simulink model "RefModel_SensorFault"  (R2020a)
settings: Solver=ode1  StartTime=0.0  StopTime=10.0  FixedStep=Ts_SensorFault.Ts_base  RelTol=1e-3
settings Model: Creator=sl  LastModifiedBy=Administrator
settings OptimizationCC: DefaultParameterBehavior=Inlined  EnhancedBackFolding=on  PassReuseOutputArgsAs=Individual arguments  ZeroExternalMemoryAtStartup=off  ZeroInternalMemoryAtStartup=off  OptimizeBlockOrder=speed  DifferentSizesBufferReuse=on  OptimizationCustomize=off  EfficientTunableParamExpr=on
settings DebuggingCC: InheritedTsInSrcMsg=none  ParameterPrecisionLossMsg=none  ParameterTunabilityLossMsg=error  UnconnectedInputMsg=none  UnconnectedOutputMsg=none  UnconnectedLineMsg=none
settings HardwareCC: ProdBitPerPointer=32  ProdBitPerSizeT=32  ProdBitPerPtrDiffT=32  ProdLargestAtomicInteger=Long  ProdLargestAtomicFloat=Double  ProdWordSize=32  ProdHWDeviceType=ARM Compatible->ARM Cortex
settings ModelReferenceCC: ModelReferenceNumInstancesAllowed=Single
settings SFSimCC: MATLABDynamicMemAlloc=off
settings RTWCC: SystemTargetFile=ert.tlc  TemplateMakefile=ert_default_tmf  GenerateReport=on  IncludeHyperlinkInReport=on  LaunchReport=on  GenerateTraceInfo=on  GenerateTraceReport=on  GenerateTraceReportSl=on  GenerateTraceReportSf=on  GenerateTraceReportEml=on
settings CodeAppCC: ForceParamTrailComments=on  IgnoreCustomStorageClasses=off  MaxIdLength=48  OperatorAnnotations=on  SimulinkDataObjDesc=on  SFDataObjDesc=on  InsertBlockDesc=on
settings ERTTargetCC: TargetLangStandard=C99 (ISO)  GenerateSampleERTMain=on  LogVarNameModifier=none  SupportVariableSizeSignals=on  InlinedParameterPlacement=NonHierarchical  ERTCustomFileTemplate=example_file_process.tlc

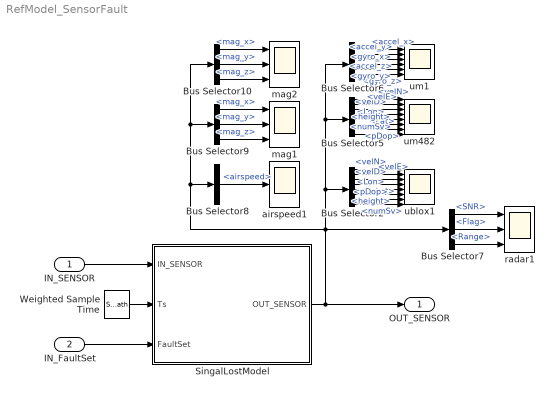
== system RefModel_SensorFault ==
  IN_SENSOR : Inport  OutDataTypeStr=Bus: BUS_SENSOR  BusOutputAsStruct=on
  IN_FaultSet : Inport  Port=2  OutDataTypeStr=Bus: BUS_SENSORFAULT_IN  BusOutputAsStruct=on
  Bus Selector10 : BusSelector  OutputSignals=mag2.mag_x,mag2.mag_y,mag2.mag_z
  Bus Selector2 : BusSelector  OutputSignals=ublox1.velN,ublox1.velE,ublox1.velD,ublox1.Lat,ublox1.Lon,ublox1.height,ublox1.pDop,ublox1.numSv
  Bus Selector5 : BusSelector  OutputSignals=um482.velN,um482.velE,um482.velD,um482.Lat,um482.Lon,um482.height,um482.pDop,um482.numSv
  Bus Selector6 : BusSelector  OutputSignals=IMU1.accel_x,IMU1.accel_y,IMU1.accel_z,IMU1.gyro_x,IMU1.gyro_y,IMU1.gyro_z
  Bus Selector7 : BusSelector  OutputSignals=radar1.SNR,radar1.Flag,radar1.Range
  Bus Selector8 : BusSelector  OutputSignals=airspeed1.airspeed
  Bus Selector9 : BusSelector  OutputSignals=mag1.mag_x,mag1.mag_y,mag1.mag_z
  SingalLostModel : Stateflow chart  TreatAsAtomicUnit=on
  Weighted Sample Time : SampleTimeMath  TsampMathOp=Ts Only
  airspeed1 : Scope
  mag1 : Scope  NumInputPorts=3
  mag2 : Scope  NumInputPorts=3
  radar1 : Scope  NumInputPorts=3
  ublox1 : Scope  NumInputPorts=8
  um1 : Scope  NumInputPorts=6
  um482 : Scope  NumInputPorts=8
  OUT_SENSOR : Outport  OutDataTypeStr=Bus: BUS_SENSOR  BusOutputAsStruct=on
  wires:
  Weighted Sample Time/1 -> SingalLostModel/2(Ts)
  IN_FaultSet/1 -> SingalLostModel/3(FaultSet)
  IN_SENSOR/1 -> SingalLostModel/1(IN_SENSOR)
  Bus Selector9/3 -> mag1/3  "<mag_z>"
  Bus Selector6/6 -> um1/6  "<gyro_z>"
  Bus Selector5/5 -> um482/5  "<Lon>"
  SingalLostModel/1(OUT_SENSOR) -> OUT_SENSOR/1, Bus Selector6/1, Bus Selector5/1, Bus Selector2/1, Bus Selector7/1, Bus Selector10/1, Bus Selector9/1, Bus Selector8/1
  Bus Selector6/4 -> um1/4  "<gyro_x>"
  Bus Selector6/2 -> um1/2  "<accel_y>"
  Bus Selector6/5 -> um1/5  "<gyro_y>"
  Bus Selector7/2 -> radar1/2  "<Flag>"
  Bus Selector5/3 -> um482/3  "<velD>"
  Bus Selector5/1 -> um482/1  "<velN>"
  Bus Selector5/4 -> um482/4  "<Lat>"
  Bus Selector5/8 -> um482/8  "<numSv>"
  Bus Selector7/3 -> radar1/3  "<Range>"
  Bus Selector5/7 -> um482/7  "<pDop>"
  Bus Selector2/1 -> ublox1/1  "<velN>"
  Bus Selector2/3 -> ublox1/3  "<velD>"
  Bus Selector2/4 -> ublox1/4  "<Lat>"
  Bus Selector6/1 -> um1/1  "<accel_x>"
  Bus Selector2/5 -> ublox1/5  "<Lon>"
  Bus Selector5/6 -> um482/6  "<height>"
  Bus Selector2/6 -> ublox1/6  "<height>"
  Bus Selector5/2 -> um482/2  "<velE>"
  Bus Selector2/8 -> ublox1/8  "<numSv>"
  Bus Selector2/2 -> ublox1/2  "<velE>"
  Bus Selector8/1 -> airspeed1/1  "<airspeed>"
  Bus Selector10/1 -> mag2/1  "<mag_x>"
  Bus Selector9/2 -> mag1/2  "<mag_y>"
  Bus Selector10/2 -> mag2/2  "<mag_y>"
  Bus Selector7/1 -> radar1/1  "<SNR>"
  Bus Selector6/3 -> um1/3  "<accel_z>"
  Bus Selector9/1 -> mag1/1  "<mag_x>"
  Bus Selector2/7 -> ublox1/7  "<pDop>"
  Bus Selector10/3 -> mag2/3  "<mag_z>"

== stateflow chart RefModel_SensorFault/SingalLostModel ==
  settings: executeAtInitialization=1
  state Others [parallel]
    settings: executionOrder=1
    state Normal
      du:
      OUT_SENSOR.time = IN_SENSOR.time;
    (default) -> Others.Normal
  state mag1 [parallel]
    en,du:
    sensorLocal = FaultSet.mag1;
    sensorDataLocal = IN_SENSOR.mag1;
    settings: executionOrder=9
    state Normal
      en:
      du:
      OUT_SENSOR.mag1 = sensorDataLocal;
    state Abnormal
      state SignalStuck
        % 信号保持最后有效值
        en:
        du:
      state SignalZero
        % 信号置零
        en,du:
        OUT_SENSOR.mag1 = setZero_mag(sensorDataLocal);
      state SignalDegrade
        % 信号精度降低
        en,du:
        OUT_SENSOR.mag1 = setDegrade_mag(sensorDataLocal);
      state SignalJump
        % 信号跳变
        en:
        tempJumpVal = 0.2*rand(1,3);
        on every((25+15*rand(1))/Ts,tick):
        tempJumpVal = 0.2*rand(1,3);
        du:
        OUT_SENSOR.mag1 = setJump_mag(sensorDataLocal,tempJumpVal);
      (default) -> mag1.Abnormal.SignalStuck
      (junction 486) -> mag1.Abnormal.SignalStuck : [whereToGo(sensorLocal) == ENUM_Fault.SingalStuck]
      (junction 488) -> (junction 486) [order 2]
      mag1.Abnormal.SignalStuck -> (junction 487) : [whereToGo(sensorLocal) ~= ENUM_Fault.SingalStuck]
      (junction 487) -> (junction 489)
      (junction 488) -> mag1.Abnormal.SignalZero [order 1] : [whereToGo(sensorLocal) == ENUM_Fault.SignalZero]
      (junction 490) -> (junction 488) [order 2]
      mag1.Abnormal.SignalZero -> (junction 489) : [whereToGo(sensorLocal) ~= ENUM_Fault.SignalZero]
      (junction 489) -> (junction 491)
      (junction 490) -> mag1.Abnormal.SignalDegrade [order 1] : [whereToGo(sensorLocal) == ENUM_Fault.SignalDegrade]
      (junction 492) -> (junction 490) [order 2]
      mag1.Abnormal.SignalDegrade -> (junction 491) : [whereToGo(sensorLocal) ~= ENUM_Fault.SignalDegrade]
      (junction 491) -> (junction 493)
      (junction 492) -> mag1.Abnormal.SignalJump [order 1] : [whereToGo(sensorLocal) == ENUM_Fault.SignalJump]
      (junction 495) -> (junction 492)
      mag1.Abnormal.SignalJump -> (junction 493) : [whereToGo(sensorLocal) ~= ENUM_Fault.SignalJump]
      (junction 493) -> (junction 494)
      (junction 494) -> (junction 495)
    (default) -> mag1.Normal
    mag1.Normal -> mag1.Abnormal : [whereToGo(sensorLocal) ~= ENUM_Fault.SignalNormal]
    mag1.Abnormal -> mag1.Normal : [whereToGo(sensorLocal) ==ENUM_Fault.SignalNormal]
  state mag2 [parallel]
    en,du:
    sensorLocal = FaultSet.mag2;
    sensorDataLocal = IN_SENSOR.mag2;
    settings: executionOrder=10
    state Normal
      en:
      du:
      OUT_SENSOR.mag2 = sensorDataLocal;
    state Abnormal
      state SignalStuck
        % 信号保持最后有效值
        en:
        du:
      state SignalZero
        % 信号置零
        en,du:
        OUT_SENSOR.mag2 = setZero_mag(sensorDataLocal);
      state SignalDegrade
        % 信号精度降低
        en,du:
        OUT_SENSOR.mag2 = setDegrade_mag(sensorDataLocal);
      state SignalJump
        % 信号跳变
        en:
        tempJumpVal = 0.2*rand(1,3);
        on every((25+15*rand(1))/Ts,tick):
        tempJumpVal = 0.2*rand(1,3);
        du:
        OUT_SENSOR.mag2 = setJump_mag(sensorDataLocal,tempJumpVal);
      (default) -> mag2.Abnormal.SignalStuck
      (junction 540) -> mag2.Abnormal.SignalStuck : [whereToGo(sensorLocal) == ENUM_Fault.SingalStuck]
      (junction 542) -> (junction 540) [order 2]
      mag2.Abnormal.SignalStuck -> (junction 541) : [whereToGo(sensorLocal) ~= ENUM_Fault.SingalStuck]
      (junction 541) -> (junction 543)
      (junction 542) -> mag2.Abnormal.SignalZero [order 1] : [whereToGo(sensorLocal) == ENUM_Fault.SignalZero]
      (junction 544) -> (junction 542) [order 2]
      mag2.Abnormal.SignalZero -> (junction 543) : [whereToGo(sensorLocal) ~= ENUM_Fault.SignalZero]
      (junction 543) -> (junction 545)
      (junction 544) -> mag2.Abnormal.SignalDegrade [order 1] : [whereToGo(sensorLocal) == ENUM_Fault.SignalDegrade]
      (junction 546) -> (junction 544) [order 2]
      mag2.Abnormal.SignalDegrade -> (junction 545) : [whereToGo(sensorLocal) ~= ENUM_Fault.SignalDegrade]
      (junction 545) -> (junction 547)
      (junction 546) -> mag2.Abnormal.SignalJump [order 1] : [whereToGo(sensorLocal) == ENUM_Fault.SignalJump]
      (junction 549) -> (junction 546)
      mag2.Abnormal.SignalJump -> (junction 547) : [whereToGo(sensorLocal) ~= ENUM_Fault.SignalJump]
      (junction 547) -> (junction 548)
      (junction 548) -> (junction 549)
    (default) -> mag2.Normal
    mag2.Normal -> mag2.Abnormal : [whereToGo(sensorLocal) ~= ENUM_Fault.SignalNormal]
    mag2.Abnormal -> mag2.Normal : [whereToGo(sensorLocal) ==ENUM_Fault.SignalNormal]
  state radar1 [parallel]
    en,du:
    sensorLocal = FaultSet.radar1;
    sensorDataLocal = IN_SENSOR.radar1;
    settings: executionOrder=7
    state Normal
      en:
      du:
      OUT_SENSOR.radar1 = sensorDataLocal;
    state Abnormal
      state SignalStuck
        % 信号保持最后有效值
        en:
        du:
      state SignalZero
        % 信号置零
        en,du:
        OUT_SENSOR.radar1 = setZero_radar(sensorDataLocal);
      state SignalDegrade
        % 信号精度降低
        en,du:
        OUT_SENSOR.radar1 = setDegrade_radar(sensorDataLocal);
      state SignalJump
        % 信号跳变
        en:
        tempJumpVal = 20*rand(1);
        on every((20+5*rand(1))/Ts,tick):
        tempJumpVal = 20*rand(1);
        on every(2,tick):
        OUT_SENSOR.radar1.Range = ...
        max(0,single(0.2*randn(1) + tempJumpVal));
      (default) -> radar1.Abnormal.SignalStuck
      (junction 335) -> radar1.Abnormal.SignalStuck : [whereToGo(sensorLocal) == ENUM_Fault.SingalStuck]
      (junction 337) -> (junction 335) [order 2]
      radar1.Abnormal.SignalStuck -> (junction 336) : [whereToGo(sensorLocal) ~= ENUM_Fault.SingalStuck]
      (junction 336) -> (junction 338)
      (junction 337) -> radar1.Abnormal.SignalZero [order 1] : [whereToGo(sensorLocal) == ENUM_Fault.SignalZero]
      (junction 339) -> (junction 337) [order 2]
      radar1.Abnormal.SignalZero -> (junction 338) : [whereToGo(sensorLocal) ~= ENUM_Fault.SignalZero]
      (junction 338) -> (junction 340)
      (junction 339) -> radar1.Abnormal.SignalDegrade [order 1] : [whereToGo(sensorLocal) == ENUM_Fault.SignalDegrade]
      (junction 341) -> (junction 339) [order 2]
      radar1.Abnormal.SignalDegrade -> (junction 340) : [whereToGo(sensorLocal) ~= ENUM_Fault.SignalDegrade]
      (junction 340) -> (junction 342)
      (junction 341) -> radar1.Abnormal.SignalJump [order 1] : [whereToGo(sensorLocal) == ENUM_Fault.SignalJump]
      (junction 344) -> (junction 341)
      radar1.Abnormal.SignalJump -> (junction 342) : [whereToGo(sensorLocal) ~= ENUM_Fault.SignalJump]
      (junction 342) -> (junction 343)
      (junction 343) -> (junction 344)
    (default) -> radar1.Normal
    radar1.Normal -> radar1.Abnormal : [whereToGo(sensorLocal) ~= ENUM_Fault.SignalNormal]
    radar1.Abnormal -> radar1.Normal : [whereToGo(sensorLocal) ==ENUM_Fault.SignalNormal]
  state airspeed1 [parallel]
    en,du:
    sensorLocal = FaultSet.airspeed1;
    sensorDataLocal = IN_SENSOR.airspeed1;
    settings: executionOrder=8
    state Normal
      en:
      du:
      OUT_SENSOR.airspeed1 = sensorDataLocal;
    state Abnormal
      state SignalStuck
        % 信号保持最后有效值
        en:
        du:
      state SignalZero
        % 信号置零
        en,du:
        OUT_SENSOR.airspeed1 = setZero_airspeed(sensorDataLocal);
      state SignalDegrade
        % 信号精度降低
        en,du:
        OUT_SENSOR.airspeed1 = setDegrade_airspeed(sensorDataLocal);
      state SignalJump
        % 信号跳变
        en:
        tempJumpVal = max(0.3,0.8*rand(1));
        on every((20+5*rand(1))/Ts,tick):
        tempJumpVal = max(0.3,0.8*rand(1));
        on every(2,tick):
        OUT_SENSOR.airspeed1.airspeed = ...
        tempJumpVal*IN_SENSOR.airspeed1.airspeed;
      (default) -> airspeed1.Abnormal.SignalStuck
      (junction 433) -> airspeed1.Abnormal.SignalStuck : [whereToGo(sensorLocal) == ENUM_Fault.SingalStuck]
      (junction 435) -> (junction 433) [order 2]
      airspeed1.Abnormal.SignalStuck -> (junction 434) : [whereToGo(sensorLocal) ~= ENUM_Fault.SingalStuck]
      (junction 434) -> (junction 436)
      (junction 435) -> airspeed1.Abnormal.SignalZero [order 1] : [whereToGo(sensorLocal) == ENUM_Fault.SignalZero]
      (junction 437) -> (junction 435) [order 2]
      airspeed1.Abnormal.SignalZero -> (junction 436) : [whereToGo(sensorLocal) ~= ENUM_Fault.SignalZero]
      (junction 436) -> (junction 438)
      (junction 437) -> airspeed1.Abnormal.SignalDegrade [order 1] : [whereToGo(sensorLocal) == ENUM_Fault.SignalDegrade]
      (junction 439) -> (junction 437) [order 2]
      airspeed1.Abnormal.SignalDegrade -> (junction 438) : [whereToGo(sensorLocal) ~= ENUM_Fault.SignalDegrade]
      (junction 438) -> (junction 440)
      (junction 439) -> airspeed1.Abnormal.SignalJump [order 1] : [whereToGo(sensorLocal) == ENUM_Fault.SignalJump]
      (junction 442) -> (junction 439)
      airspeed1.Abnormal.SignalJump -> (junction 440) : [whereToGo(sensorLocal) ~= ENUM_Fault.SignalJump]
      (junction 440) -> (junction 441)
      (junction 441) -> (junction 442)
    (default) -> airspeed1.Normal
    airspeed1.Normal -> airspeed1.Abnormal : [whereToGo(sensorLocal) ~= ENUM_Fault.SignalNormal]
    airspeed1.Abnormal -> airspeed1.Normal : [whereToGo(sensorLocal) ==ENUM_Fault.SignalNormal]
  state baro1 [parallel]
    en,du:
    sensorLocal = FaultSet.baro1;
    sensorDataLocal = IN_SENSOR.baro1;
    settings: executionOrder=11
    state Normal
      en:
      du:
      OUT_SENSOR.baro1 = sensorDataLocal;
    state Abnormal
      state SignalStuck
        % 信号保持最后有效值
        en:
        du:
      state SignalZero
        % 信号置零
        en,du:
        OUT_SENSOR.baro1 = setZero_baro(sensorDataLocal);
      state SignalDegrade
        % 信号精度降低
        en,du:
        OUT_SENSOR.baro1 = setDegrade_baro(sensorDataLocal);
      state SignalJump
        % 信号跳变
        en:
        tempJumpVal = 20*rand(1);
        on every((20+5*rand(1))/Ts,tick):
        tempJumpVal = 20*rand(1);
        on every(2,tick):
        OUT_SENSOR.baro1.alt_baro = ...
        max(0,single(0.2*randn(1) + tempJumpVal));
      (default) -> baro1.Abnormal.SignalStuck
      (junction 584) -> baro1.Abnormal.SignalStuck : [whereToGo(sensorLocal) == ENUM_Fault.SingalStuck]
      (junction 586) -> (junction 584) [order 2]
      baro1.Abnormal.SignalStuck -> (junction 585) : [whereToGo(sensorLocal) ~= ENUM_Fault.SingalStuck]
      (junction 585) -> (junction 587)
      (junction 586) -> baro1.Abnormal.SignalZero [order 1] : [whereToGo(sensorLocal) == ENUM_Fault.SignalZero]
      (junction 588) -> (junction 586) [order 2]
      baro1.Abnormal.SignalZero -> (junction 587) : [whereToGo(sensorLocal) ~= ENUM_Fault.SignalZero]
      (junction 587) -> (junction 589)
      (junction 588) -> baro1.Abnormal.SignalDegrade [order 1] : [whereToGo(sensorLocal) == ENUM_Fault.SignalDegrade]
      (junction 590) -> (junction 588) [order 2]
      baro1.Abnormal.SignalDegrade -> (junction 589) : [whereToGo(sensorLocal) ~= ENUM_Fault.SignalDegrade]
      (junction 589) -> (junction 591)
      (junction 590) -> baro1.Abnormal.SignalJump [order 1] : [whereToGo(sensorLocal) == ENUM_Fault.SignalJump]
      (junction 593) -> (junction 590)
      baro1.Abnormal.SignalJump -> (junction 591) : [whereToGo(sensorLocal) ~= ENUM_Fault.SignalJump]
      (junction 591) -> (junction 592)
      (junction 592) -> (junction 593)
    (default) -> baro1.Normal
    baro1.Normal -> baro1.Abnormal : [whereToGo(sensorLocal) ~= ENUM_Fault.SignalNormal]
    baro1.Abnormal -> baro1.Normal : [whereToGo(sensorLocal) ==ENUM_Fault.SignalNormal]
  state IMU1 [parallel]
    en,du:
    sensorLocal = FaultSet.IMU1;
    sensorDataLocal = IN_SENSOR.IMU1;
    settings: executionOrder=4
    state Normal
      en:
      du:
      OUT_SENSOR.IMU1 = sensorDataLocal;
    state Abnormal
      state SignalStuck
        % 信号保持最后有效值
        en:
        du:
      state SignalZero
        % 信号置零
        en,du:
        OUT_SENSOR.IMU1 = setZero_IMU(sensorDataLocal);
      state SignalDegrade
        % 信号精度降低
        en,du:
        OUT_SENSOR.IMU1 = setDegrade_IMU(sensorDataLocal);
      state SignalJump
        % 信号跳变
        du:
        OUT_SENSOR.IMU1 = sensorDataLocal;
        on every((2+5*rand(1))/Ts,tick):
        OUT_SENSOR.IMU1 = setJump_IMU(sensorDataLocal);
      (default) -> IMU1.Abnormal.SignalStuck
      (junction 197) -> IMU1.Abnormal.SignalStuck : [whereToGo(sensorLocal) == ENUM_Fault.SingalStuck]
      (junction 199) -> (junction 197) [order 2]
      IMU1.Abnormal.SignalStuck -> (junction 198) : [whereToGo(sensorLocal) ~= ENUM_Fault.SingalStuck]
      (junction 198) -> (junction 200)
      (junction 199) -> IMU1.Abnormal.SignalZero [order 1] : [whereToGo(sensorLocal) == ENUM_Fault.SignalZero]
      (junction 201) -> (junction 199) [order 2]
      IMU1.Abnormal.SignalZero -> (junction 200) : [whereToGo(sensorLocal) ~= ENUM_Fault.SignalZero]
      (junction 200) -> (junction 202)
      (junction 201) -> IMU1.Abnormal.SignalDegrade [order 1] : [whereToGo(sensorLocal) == ENUM_Fault.SignalDegrade]
      (junction 203) -> (junction 201) [order 2]
      IMU1.Abnormal.SignalDegrade -> (junction 202) : [whereToGo(sensorLocal) ~= ENUM_Fault.SignalDegrade]
      (junction 202) -> (junction 204)
      (junction 203) -> IMU1.Abnormal.SignalJump [order 1] : [whereToGo(sensorLocal) == ENUM_Fault.SignalJump]
      (junction 206) -> (junction 203)
      IMU1.Abnormal.SignalJump -> (junction 204) : [whereToGo(sensorLocal) ~= ENUM_Fault.SignalJump]
      (junction 204) -> (junction 205)
      (junction 205) -> (junction 206)
    (default) -> IMU1.Normal
    IMU1.Normal -> IMU1.Abnormal : [whereToGo(sensorLocal) ~= ENUM_Fault.SignalNormal]
    IMU1.Abnormal -> IMU1.Normal : [whereToGo(sensorLocal) ==ENUM_Fault.SignalNormal]
  state IMU2 [parallel]
    en,du:
    sensorLocal = FaultSet.IMU2;
    sensorDataLocal = IN_SENSOR.IMU2;
    settings: executionOrder=5
    state Normal
      en:
      du:
      OUT_SENSOR.IMU2 = sensorDataLocal;
    state Abnormal
      state SignalStuck
        % 信号保持最后有效值
        en:
        du:
      state SignalZero
        % 信号置零
        en,du:
        OUT_SENSOR.IMU2 = setZero_IMU(sensorDataLocal);
      state SignalDegrade
        % 信号精度降低
        en,du:
        OUT_SENSOR.IMU2 = setDegrade_IMU(sensorDataLocal);
      state SignalJump
        % 信号跳变
        du:
        OUT_SENSOR.IMU2 = sensorDataLocal;
        on every((2+5*rand(1))/Ts,tick):
        OUT_SENSOR.IMU2 = setJump_IMU(sensorDataLocal);
      (default) -> IMU2.Abnormal.SignalStuck
      (junction 249) -> IMU2.Abnormal.SignalStuck : [whereToGo(sensorLocal) == ENUM_Fault.SingalStuck]
      (junction 251) -> (junction 249) [order 2]
      IMU2.Abnormal.SignalStuck -> (junction 250) : [whereToGo(sensorLocal) ~= ENUM_Fault.SingalStuck]
      (junction 250) -> (junction 252)
      (junction 251) -> IMU2.Abnormal.SignalZero [order 1] : [whereToGo(sensorLocal) == ENUM_Fault.SignalZero]
      (junction 253) -> (junction 251) [order 2]
      IMU2.Abnormal.SignalZero -> (junction 252) : [whereToGo(sensorLocal) ~= ENUM_Fault.SignalZero]
      (junction 252) -> (junction 254)
      (junction 253) -> IMU2.Abnormal.SignalDegrade [order 1] : [whereToGo(sensorLocal) == ENUM_Fault.SignalDegrade]
      (junction 255) -> (junction 253) [order 2]
      IMU2.Abnormal.SignalDegrade -> (junction 254) : [whereToGo(sensorLocal) ~= ENUM_Fault.SignalDegrade]
      (junction 254) -> (junction 256)
      (junction 255) -> IMU2.Abnormal.SignalJump [order 1] : [whereToGo(sensorLocal) == ENUM_Fault.SignalJump]
      (junction 258) -> (junction 255)
      IMU2.Abnormal.SignalJump -> (junction 256) : [whereToGo(sensorLocal) ~= ENUM_Fault.SignalJump]
      (junction 256) -> (junction 257)
      (junction 257) -> (junction 258)
    (default) -> IMU2.Normal
    IMU2.Normal -> IMU2.Abnormal : [whereToGo(sensorLocal) ~= ENUM_Fault.SignalNormal]
    IMU2.Abnormal -> IMU2.Normal : [whereToGo(sensorLocal) ==ENUM_Fault.SignalNormal]
  state IMU3 [parallel]
    en,du:
    sensorLocal = FaultSet.IMU3;
    sensorDataLocal = IN_SENSOR.IMU3;
    settings: executionOrder=6
    state Normal
      en:
      du:
      OUT_SENSOR.IMU3 = sensorDataLocal;
    state Abnormal
      state SignalStuck
        % 信号保持最后有效值
        en:
        du:
      state SignalZero
        % 信号置零
        en,du:
        OUT_SENSOR.IMU3 = setZero_IMU(sensorDataLocal);
      state SignalDegrade
        % 信号精度降低
        en,du:
        OUT_SENSOR.IMU3 = setDegrade_IMU(sensorDataLocal);
      state SignalJump
        % 信号跳变
        du:
        OUT_SENSOR.IMU3 = sensorDataLocal;
        on every((2+5*rand(1))/Ts,tick):
        OUT_SENSOR.IMU3 = setJump_IMU(sensorDataLocal);
      (default) -> IMU3.Abnormal.SignalStuck
      (junction 292) -> IMU3.Abnormal.SignalStuck : [whereToGo(sensorLocal) == ENUM_Fault.SingalStuck]
      (junction 294) -> (junction 292) [order 2]
      IMU3.Abnormal.SignalStuck -> (junction 293) : [whereToGo(sensorLocal) ~= ENUM_Fault.SingalStuck]
      (junction 293) -> (junction 295)
      (junction 294) -> IMU3.Abnormal.SignalZero [order 1] : [whereToGo(sensorLocal) == ENUM_Fault.SignalZero]
      (junction 296) -> (junction 294) [order 2]
      IMU3.Abnormal.SignalZero -> (junction 295) : [whereToGo(sensorLocal) ~= ENUM_Fault.SignalZero]
      (junction 295) -> (junction 297)
      (junction 296) -> IMU3.Abnormal.SignalDegrade [order 1] : [whereToGo(sensorLocal) == ENUM_Fault.SignalDegrade]
      (junction 298) -> (junction 296) [order 2]
      IMU3.Abnormal.SignalDegrade -> (junction 297) : [whereToGo(sensorLocal) ~= ENUM_Fault.SignalDegrade]
      (junction 297) -> (junction 299)
      (junction 298) -> IMU3.Abnormal.SignalJump [order 1] : [whereToGo(sensorLocal) == ENUM_Fault.SignalJump]
      (junction 301) -> (junction 298)
      IMU3.Abnormal.SignalJump -> (junction 299) : [whereToGo(sensorLocal) ~= ENUM_Fault.SignalJump]
      (junction 299) -> (junction 300)
      (junction 300) -> (junction 301)
    (default) -> IMU3.Normal
    IMU3.Normal -> IMU3.Abnormal : [whereToGo(sensorLocal) ~= ENUM_Fault.SignalNormal]
    IMU3.Abnormal -> IMU3.Normal : [whereToGo(sensorLocal) ==ENUM_Fault.SignalNormal]
  state ublox1 [parallel]
    en,du:
    sensorLocal = FaultSet.ublox1;
    sensorDataLocal = IN_SENSOR.ublox1;
    settings: executionOrder=2
    state Normal
      en:
      du:
      OUT_SENSOR.ublox1 = sensorDataLocal;
    state Abnormal
      state SignalStuck
        % 信号保持最后有效值
        en:
        du:
      state SignalZero
        % 信号置零
        en,du:
        OUT_SENSOR.ublox1 = setZero_ublox(sensorDataLocal);
      state SignalDegrade
        % 信号精度降低
        en,du:
        OUT_SENSOR.ublox1 = setDegrade_ublox(sensorDataLocal);
      state SignalJump
        % 信号跳变
        du:
        OUT_SENSOR.ublox1 = sensorDataLocal;
        % on every((2+5*rand(1))/Ts,tick):
        OUT_SENSOR.ublox1 = setJump_ublox(sensorDataLocal);
      (default) -> ublox1.Abnormal.SignalStuck
      (junction 90) -> ublox1.Abnormal.SignalStuck : [whereToGo(sensorLocal) == ENUM_Fault.SingalStuck]
      (junction 91) -> (junction 90) [order 2]
      ublox1.Abnormal.SignalStuck -> (junction 87) : [whereToGo(sensorLocal) ~= ENUM_Fault.SingalStuck]
      (junction 87) -> (junction 88)
      (junction 91) -> ublox1.Abnormal.SignalZero [order 1] : [whereToGo(sensorLocal) == ENUM_Fault.SignalZero]
      (junction 104) -> (junction 91) [order 2]
      ublox1.Abnormal.SignalZero -> (junction 88) : [whereToGo(sensorLocal) ~= ENUM_Fault.SignalZero]
      (junction 88) -> (junction 101)
      (junction 104) -> ublox1.Abnormal.SignalDegrade [order 1] : [whereToGo(sensorLocal) == ENUM_Fault.SignalDegrade]
      (junction 105) -> (junction 104) [order 2]
      ublox1.Abnormal.SignalDegrade -> (junction 101) : [whereToGo(sensorLocal) ~= ENUM_Fault.SignalDegrade]
      (junction 101) -> (junction 97)
      (junction 105) -> ublox1.Abnormal.SignalJump [order 1] : [whereToGo(sensorLocal) == ENUM_Fault.SignalJump]
      (junction 109) -> (junction 105)
      ublox1.Abnormal.SignalJump -> (junction 97) : [whereToGo(sensorLocal) ~= ENUM_Fault.SignalJump]
      (junction 97) -> (junction 108)
      (junction 108) -> (junction 109)
    (default) -> ublox1.Normal
    ublox1.Normal -> ublox1.Abnormal : [whereToGo(sensorLocal) ~= ENUM_Fault.SignalNormal]
    ublox1.Abnormal -> ublox1.Normal : [whereToGo(sensorLocal) ==ENUM_Fault.SignalNormal]
        | %after(FaultSet.ublox1.duration,sec)]
  state um482 [parallel]
    en,du:
    sensorLocal = FaultSet.um482;
    sensorDataLocal = IN_SENSOR.um482;
    settings: executionOrder=3
    state Normal
      en:
      du:
      OUT_SENSOR.um482 = sensorDataLocal;
    state Abnormal
      state SignalStuck
        % 信号保持最后有效值
        en:
        du:
      state SignalZero
        % 信号置零
        en,du:
        OUT_SENSOR.um482 = setZero_um482(sensorDataLocal);
      state SignalDegrade
        % 信号精度降低
        en,du:
        OUT_SENSOR.um482 = setDegrade_um482(sensorDataLocal);
      state SignalJump
        % 信号跳变
        du:
        OUT_SENSOR.um482 = sensorDataLocal;
        % on every((2+5*rand(1))/Ts,tick):
        OUT_SENSOR.um482 = setJump_um482(sensorDataLocal);
      (default) -> um482.Abnormal.SignalStuck
      (junction 143) -> um482.Abnormal.SignalStuck : [whereToGo(sensorLocal) == ENUM_Fault.SingalStuck]
      (junction 145) -> (junction 143) [order 2]
      um482.Abnormal.SignalStuck -> (junction 144) : [whereToGo(sensorLocal) ~= ENUM_Fault.SingalStuck]
      (junction 144) -> (junction 146)
      (junction 145) -> um482.Abnormal.SignalZero [order 1] : [whereToGo(sensorLocal) == ENUM_Fault.SignalZero]
      (junction 147) -> (junction 145) [order 2]
      um482.Abnormal.SignalZero -> (junction 146) : [whereToGo(sensorLocal) ~= ENUM_Fault.SignalZero]
      (junction 146) -> (junction 148)
      (junction 147) -> um482.Abnormal.SignalDegrade [order 1] : [whereToGo(sensorLocal) == ENUM_Fault.SignalDegrade]
      (junction 149) -> (junction 147) [order 2]
      um482.Abnormal.SignalDegrade -> (junction 148) : [whereToGo(sensorLocal) ~= ENUM_Fault.SignalDegrade]
      (junction 148) -> (junction 150)
      (junction 149) -> um482.Abnormal.SignalJump [order 1] : [whereToGo(sensorLocal) == ENUM_Fault.SignalJump]
      (junction 152) -> (junction 149)
      um482.Abnormal.SignalJump -> (junction 150) : [whereToGo(sensorLocal) ~= ENUM_Fault.SignalJump]
      (junction 150) -> (junction 151)
      (junction 151) -> (junction 152)
    (default) -> um482.Normal
    um482.Normal -> um482.Abnormal : [whereToGo(sensorLocal) ~= ENUM_Fault.SignalNormal]
    um482.Abnormal -> um482.Normal : [whereToGo(sensorLocal) ==ENUM_Fault.SignalNormal]
        | %after(FaultSet.ublox1.duration,sec)]
  data: out function_output; ublox function_input; out function_output; ublox function_input; out function_output; ublox function_input; out function_output; sensor function_input; sensorLocal local Bus: BUS_SENSORFAULT_SensorParam; sensorDataLocal local Bus: BUS_MAG; tempJumpVal local; out function_output; sensor function_input; sensorLocal local Bus: BUS_SENSORFAULT_SensorParam; sensorDataLocal local Bus: BUS_MAG; tempJumpVal local; out function_output; um482 function_input; out function_output; um482 function_input; out function_output; um482 function_input; out function_output; sensor function_input; sensorLocal local Bus: BUS_SENSORFAULT_SensorParam; sensorDataLocal local Bus: BUS_RADAR; tempJumpVal local; out function_output; sensor function_input; sensorLocal local Bus: BUS_SENSORFAULT_SensorParam; sensorDataLocal local Bus: BUS_AIRSPEED; tempJumpVal local; out function_output; sensor function_input; sensorLocal local Bus: BUS_SENSORFAULT_SensorParam; sensorDataLocal local Bus: BUS_BARO; tempJumpVal local; out function_output; imu function_input; out function_output; imu function_input; out function_output; imu function_input; out function_output; radar function_input; out function_output; radar function_input; out function_output; radar function_input; out function_output; sensor function_input; sensorLocal local Bus: BUS_SENSORFAULT_SensorParam; sensorDataLocal local Bus: BUS_IMU; out function_output; sensor function_input; sensorLocal local Bus: BUS_SENSORFAULT_SensorParam; sensorDataLocal local Bus: BUS_IMU; out function_output; sensor function_input; sensorLocal local Bus: BUS_SENSORFAULT_SensorParam; sensorDataLocal local Bus: BUS_IMU; out function_output; airspeed function_input; out function_output; airspeed function_input; out function_output; sensor function_input; sensorLocal local Bus: BUS_SENSORFAULT_SensorParam; sensorDataLocal local Bus: BUS_UBLOX; out function_output; sensor function_input; sensorLocal local Bus: BUS_SENSORFAULT_SensorParam; sensorDataLocal local Bus: BUS_UM482; out function_output; mag function_input; out function_output; mag function_input; out function_output; mag function_input; bias function_input; out function_output; baro function_input; out function_output; baro function_input; IN_SENSOR input Bus: BUS_SENSOR; OUT_SENSOR output Bus: BUS_SENSOR; Ts input; idx local; FaultSet input
  events: event_gotoAbnormal_ublox1 local FUNCTION_CALL_EVENT
  function out = setZero_ublox(ublox):
    | function out = setZero_ublox(ublox)
    | out = ublox;
    | out.velN = single(0);
    | out.velE = single(0);
    | out.velD = single(0);
    | out.Lat = double(0);
    | out.Lon = double(0);
    | out.height = single(0);
    | out.pDop = single(0);
    | out.numSv = single(0);
    | out.hAcc = single(0);
    | out.vAcc = single(0);
    | out.sAcc = single(0);
    | out.headAcc = single(0);
  function out = setDegrade_ublox(ublox):
    | function out = setDegrade_ublox(ublox)
    | out = ublox;
    | kVel = 2;
    | kPos = 5; % m
    | out.velN = out.velN*kVel*randn(1)/3;
    | out.velE = out.velE*kVel*randn(1)/3;
    | out.velD = out.velD*kVel*randn(1)/3;
    | out.Lat = out.Lat + kPos*1/111e3*randn(1)/3;
    | out.Lon = out.Lon + kPos*1/111e3*randn(1)/3;
    | out.height = out.height + kPos*randn(1)/3;
    | out.pDop = single(6);
    | out.numSv = single(9);
    | % out.hAcc = single(0);
    | % out.vAcc = single(0);
    | % out.sAcc = single(0);
    | % out.headAcc = single(0);
  function out = setJump_ublox(ublox):
    | function out = setJump_ublox(ublox)
    | out = ublox;
    | kVel = 10;
    | kPos = 20; % m
    | out.velN = out.velN+kVel*randn(1)/3;
    | out.velE = out.velE+kVel*randn(1)/3;
    | out.velD = out.velD+kVel*randn(1)/3;
    | out.Lat = out.Lat + kPos*1/111e3*randn(1)/3;
    | out.Lon = out.Lon + kPos*1/111e3*randn(1)/3;
    | out.height = out.height + kPos*randn(1)/3;
    | out.pDop = single(12);
    | out.numSv = single(6);
    | % out.hAcc = single(0);
    | % out.vAcc = single(0);
    | % out.sAcc = single(0);
    | % out.headAcc = single(0);
  function out = whereToGo(sensor):
    | function out = whereToGo(sensor)
    | out = ENUM_Fault.SignalNormal;
    | if sensor.status == ENUM_Fault.SingalStuck % stuck 1级
    |     out = ENUM_Fault.SingalStuck;
    |     return;
    | end
    | if sensor.status == ENUM_Fault.SignalZero % zero 2级
    |     out = ENUM_Fault.SignalZero;
    |     return;
    | end
    | if sensor.status == ENUM_Fault.SignalJump %
    |     out = ENUM_Fault.SignalJump;
    |     return;
    | end
    | if sensor.status == ENUM_Fault.SignalDegrade % 
    |     out = ENUM_Fault.SignalDegrade;
    |     return;
    | end
  function out = whereToGo(sensor):
    | function out = whereToGo(sensor)
    | out = ENUM_Fault.SignalNormal;
    | if sensor.status == ENUM_Fault.SingalStuck % stuck 1级
    |     out = ENUM_Fault.SingalStuck;
    |     return;
    | end
    | if sensor.status == ENUM_Fault.SignalZero % zero 2级
    |     out = ENUM_Fault.SignalZero;
    |     return;
    | end
    | if sensor.status == ENUM_Fault.SignalJump %
    |     out = ENUM_Fault.SignalJump;
    |     return;
    | end
    | if sensor.status == ENUM_Fault.SignalDegrade % 
    |     out = ENUM_Fault.SignalDegrade;
    |     return;
    | end
  function out = setZero_um482(um482):
    | function out = setZero_um482(um482)
    | out = um482;
    | out.velN = single(0);
    | out.velE = single(0);
    | out.velD = single(0);
    | out.Lat = double(0);
    | out.Lon = double(0);
    | out.height = single(0);
    | out.pDop = single(0);
    | out.numSv = single(0);
    | out.delta_lat = single(0);
    | out.delta_lon = single(0);
    | out.delta_height = single(0);
    | out.BESTPOS = int8(0);
  function out = setDegrade_um482(um482):
    | function out = setDegrade_um482(um482)
    | out = um482;
    | kVel = 2;
    | kPos = 5; % m
    | out.velN = out.velN*kVel*randn(1)/3;
    | out.velE = out.velE*kVel*randn(1)/3;
    | out.velD = out.velD*kVel*randn(1)/3;
    | out.Lat = out.Lat + kPos*1/111e3*randn(1)/3;
    | out.Lon = out.Lon + kPos*1/111e3*randn(1)/3;
    | out.height = out.height + kPos*randn(1)/3;
    | out.pDop = single(4);
    | out.numSv = single(18);
    | out.delta_lat = single(5);
    | out.delta_lon = single(10);
    | out.delta_height = single(6);
    | out.BESTPOS = int8(16);
  function out = setJump_um482(um482):
    | function out = setJump_um482(um482)
    | out = um482;
    | kVel = 10;
    | kPos = 20; % m
    | out.velN = out.velN+kVel*randn(1)/3;
    | out.velE = out.velE+kVel*randn(1)/3;
    | out.velD = out.velD+kVel*randn(1)/3;
    | out.Lat = out.Lat + kPos*1/111e3*randn(1)/3;
    | out.Lon = out.Lon + kPos*1/111e3*randn(1)/3;
    | out.height = out.height + kPos*randn(1)/3;
    | out.pDop = single(15);
    | out.numSv = single(12);
    | out.delta_lat = single(5);
    | out.delta_lon = single(10);
    | out.delta_height = single(6);
    | out.BESTPOS = int8(16);
  function out = whereToGo(sensor):
    | function out = whereToGo(sensor)
    | out = ENUM_Fault.SignalNormal;
    | if sensor.status == ENUM_Fault.SingalStuck % stuck 1级
    |     out = ENUM_Fault.SingalStuck;
    |     return;
    | end
    | if sensor.status == ENUM_Fault.SignalZero % zero 2级
    |     out = ENUM_Fault.SignalZero;
    |     return;
    | end
    | if sensor.status == ENUM_Fault.SignalJump %
    |     out = ENUM_Fault.SignalJump;
    |     return;
    | end
    | if sensor.status == ENUM_Fault.SignalDegrade % 
    |     out = ENUM_Fault.SignalDegrade;
    |     return;
    | end
  function out = whereToGo(sensor):
    | function out = whereToGo(sensor)
    | out = ENUM_Fault.SignalNormal;
    | if sensor.status == ENUM_Fault.SingalStuck % stuck 1级
    |     out = ENUM_Fault.SingalStuck;
    |     return;
    | end
    | if sensor.status == ENUM_Fault.SignalZero % zero 2级
    |     out = ENUM_Fault.SignalZero;
    |     return;
    | end
    | if sensor.status == ENUM_Fault.SignalJump %
    |     out = ENUM_Fault.SignalJump;
    |     return;
    | end
    | if sensor.status == ENUM_Fault.SignalDegrade % 
    |     out = ENUM_Fault.SignalDegrade;
    |     return;
    | end
  function out = whereToGo(sensor):
    | function out = whereToGo(sensor)
    | out = ENUM_Fault.SignalNormal;
    | if sensor.status == ENUM_Fault.SingalStuck % stuck 1级
    |     out = ENUM_Fault.SingalStuck;
    |     return;
    | end
    | if sensor.status == ENUM_Fault.SignalZero % zero 2级
    |     out = ENUM_Fault.SignalZero;
    |     return;
    | end
    | if sensor.status == ENUM_Fault.SignalJump %
    |     out = ENUM_Fault.SignalJump;
    |     return;
    | end
    | if sensor.status == ENUM_Fault.SignalDegrade % 
    |     out = ENUM_Fault.SignalDegrade;
    |     return;
    | end
  function out = setZero_IMU(imu):
    | function out = setZero_IMU(imu)
    | out = imu;
    | out.accel_x = single(0);
    | out.accel_y = single(0);
    | out.accel_z = single(0);
    | out.gyro_x = single(0);
    | out.gyro_y = single(0);
    | out.gyro_z = single(0);
  function out = setDegrade_IMU(imu):
    | function out = setDegrade_IMU(imu)
    | out = imu;
    | kAcc = 10; % m/s^2
    | kGyro = 10; % rad/s
    | out.accel_x = out.accel_x*kAcc*randn(1)/3;
    | out.accel_y = out.accel_y*kAcc*randn(1)/3;
    | out.accel_z = out.accel_z*kAcc*randn(1)/3;
    | out.gyro_x = out.gyro_x*kGyro*randn(1)/3;
    | out.gyro_y = out.gyro_y*kGyro*randn(1)/3;
    | out.gyro_z = out.gyro_z*kGyro*randn(1)/3;
  function out = setJump_IMU(imu):
    | function out = setJump_IMU(imu)
    | out = imu;
    | kAcc = 10; % m/s^2
    | kGyro = 10; % rad/s
    | out.accel_x = out.accel_x*kAcc*randn(1)/3;
    | out.accel_y = out.accel_y*kAcc*randn(1)/3;
    | out.accel_z = out.accel_z*kAcc*randn(1)/3;
    | out.gyro_x = out.gyro_x*kGyro*randn(1)/3;
    | out.gyro_y = out.gyro_y*kGyro*randn(1)/3;
    | out.gyro_z = out.gyro_z*kGyro*randn(1)/3;
  function out = setZero_radar(radar):
    | function out = setZero_radar(radar)
    | out = radar;
    | out.SNR = single(0);
    | out.Flag = single(0);
    | out.Range = single(0);
  function out = setDegrade_radar(radar):
    | function out = setDegrade_radar(radar)
    | out = radar;
    | kRange = 10; %
    | % out.SNR = single(0);
    | % out.Flag = single(0);
    | out.Range = out.Range*kRange*randn(1)/3;
  function out = setJump_radar(radar):
    | function out = setJump_radar(radar)
    | out = radar;
    | % out.SNR = single(0);
    | % out.Flag = single(0);
    | out.Range = 0.2*randn(1) + tempJumpVal;
  function out = whereToGo(sensor):
    | function out = whereToGo(sensor)
    | out = ENUM_Fault.SignalNormal;
    | if sensor.status == ENUM_Fault.SingalStuck % stuck 1级
    |     out = ENUM_Fault.SingalStuck;
    |     return;
    | end
    | if sensor.status == ENUM_Fault.SignalZero % zero 2级
    |     out = ENUM_Fault.SignalZero;
    |     return;
    | end
    | if sensor.status == ENUM_Fault.SignalJump %
    |     out = ENUM_Fault.SignalJump;
    |     return;
    | end
    | if sensor.status == ENUM_Fault.SignalDegrade % 
    |     out = ENUM_Fault.SignalDegrade;
    |     return;
    | end
  function out = whereToGo(sensor):
    | function out = whereToGo(sensor)
    | out = ENUM_Fault.SignalNormal;
    | if sensor.status == ENUM_Fault.SingalStuck % stuck 1级
    |     out = ENUM_Fault.SingalStuck;
    |     return;
    | end
    | if sensor.status == ENUM_Fault.SignalZero % zero 2级
    |     out = ENUM_Fault.SignalZero;
    |     return;
    | end
    | if sensor.status == ENUM_Fault.SignalJump %
    |     out = ENUM_Fault.SignalJump;
    |     return;
    | end
    | if sensor.status == ENUM_Fault.SignalDegrade % 
    |     out = ENUM_Fault.SignalDegrade;
    |     return;
    | end
  function out = whereToGo(sensor):
    | function out = whereToGo(sensor)
    | out = ENUM_Fault.SignalNormal;
    | if sensor.status == ENUM_Fault.SingalStuck % stuck 1级
    |     out = ENUM_Fault.SingalStuck;
    |     return;
    | end
    | if sensor.status == ENUM_Fault.SignalZero % zero 2级
    |     out = ENUM_Fault.SignalZero;
    |     return;
    | end
    | if sensor.status == ENUM_Fault.SignalJump %
    |     out = ENUM_Fault.SignalJump;
    |     return;
    | end
    | if sensor.status == ENUM_Fault.SignalDegrade % 
    |     out = ENUM_Fault.SignalDegrade;
    |     return;
    | end
  function out = setZero_airspeed(airspeed):
    | function out = setZero_airspeed(airspeed)
    | out = airspeed;
    | out.airspeed = single(0);
  function out = setDegrade_airspeed(airspeed):
    | function out = setDegrade_airspeed(airspeed)
    | out = airspeed;
    | K = 2;
    | out.airspeed = out.airspeed*K*randn(1)/3;
  function out = whereToGo(sensor):
    | function out = whereToGo(sensor)
    | out = ENUM_Fault.SignalNormal;
    | if sensor.status == ENUM_Fault.SingalStuck % stuck 1级
    |     out = ENUM_Fault.SingalStuck;
    |     return;
    | end
    | if sensor.status == ENUM_Fault.SignalZero % zero 2级
    |     out = ENUM_Fault.SignalZero;
    |     return;
    | end
    | if sensor.status == ENUM_Fault.SignalJump %
    |     out = ENUM_Fault.SignalJump;
    |     return;
    | end
    | if sensor.status == ENUM_Fault.SignalDegrade % 
    |     out = ENUM_Fault.SignalDegrade;
    |     return;
    | end
  function out = whereToGo(sensor):
    | function out = whereToGo(sensor)
    | out = ENUM_Fault.SignalNormal;
    | if sensor.status == ENUM_Fault.SingalStuck % stuck 1级
    |     out = ENUM_Fault.SingalStuck;
    |     return;
    | end
    | if sensor.status == ENUM_Fault.SignalZero % zero 2级
    |     out = ENUM_Fault.SignalZero;
    |     return;
    | end
    | if sensor.status == ENUM_Fault.SignalJump %
    |     out = ENUM_Fault.SignalJump;
    |     return;
    | end
    | if sensor.status == ENUM_Fault.SignalDegrade % 
    |     out = ENUM_Fault.SignalDegrade;
    |     return;
    | end
  function out = setDegrade_mag(mag):
    | function out = setDegrade_mag(mag)
    | out = mag;
    | K = 1.5;
    | out.mag_x = out.mag_x*K*randn(1)/3;
    | out.mag_y = out.mag_y*K*randn(1)/3;
    | out.mag_z = out.mag_z*K*randn(1)/3;
  function out = setZero_mag(mag):
    | function out = setZero_mag(mag)
    | out = mag;
    | out.mag_x = single(0);
    | out.mag_y = single(0);
    | out.mag_z = single(0);
  function out = setJump_mag(mag,bias):
    | function out = setJump_mag(mag,bias)
    | out = mag;
    | out.mag_x = out.mag_x + bias(1);
    | out.mag_y = out.mag_y + bias(2);
    | out.mag_z = out.mag_z + bias(3);
  function out = setZero_baro(baro):
    | function out = setZero_baro(baro)
    | out = baro;
    | out.alt_baro = single(0);
  function out = setDegrade_baro(baro):
    | function out = setDegrade_baro(baro)
    | out = baro;
    | K = 10; %
    | out.alt_baro = out.alt_baro*K*randn(1)/3;
